simulink model "Active_Suspension_LQR"  (Simulink 7.3)
settings: Solver=ode3  StartTime=0.0  StopTime=50  FixedStep=0.005  RelTol=1e-3
values from neighbouring files (symbols this model uses):
  A = [0,0,-ks/mb,ks/mb,0;0,0,ks/mw,(-kt-ks)/mw,kt/mw;1,0,0,0,0;0,1,0,0,0;0,0,0,0,-2*pi*f0]    [GA_LQR.m]
  B = [1/mb;-1/mw;0;0;0]    [GA_LQR.m]
  C = eye(size(A,1))    [GA_LQR.m]
  D = zeros(size(A,1),size(B,2))    [GA_LQR.m]
  G = [0;0;0;0;2*pi*sqrt(G0*u)]    [GA_LQR.m]
undefined symbols (not defined in the file or in its folder): K
settings Model: Creator=tongji_HEV  LastModifiedBy=tongji_HEV

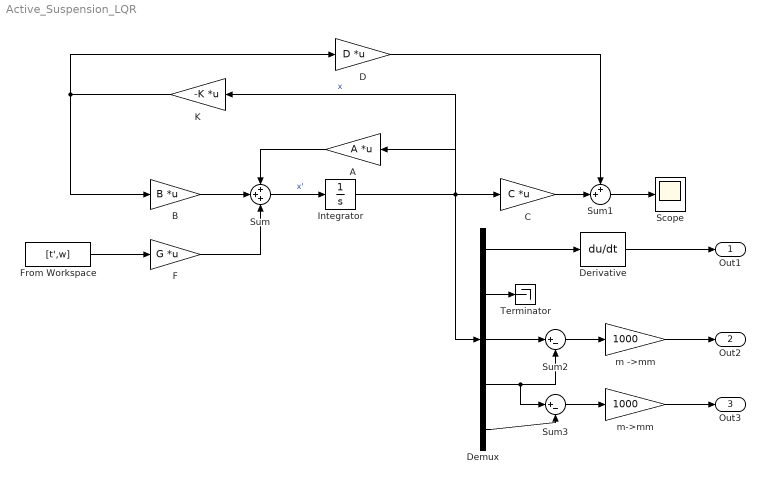
== system Active_Suspension_LQR ==
  A : Gain  Gain=A  Multiplication=Matrix(K*u)  ParameterDataType=fixdt(1, 16)  ParameterScaling=2^0  OutDataType=fixdt(1, 16)  OutScaling=2^0
  B : Gain  Gain=B  Multiplication=Matrix(K*u)  ParameterDataType=fixdt(1, 16)  ParameterScaling=2^0  OutDataType=fixdt(1, 16)  OutScaling=2^0
  C : Gain  Gain=C  Multiplication=Matrix(K*u)  ParameterDataType=fixdt(1, 16)  ParameterScaling=2^0  OutDataType=fixdt(1, 16)  OutScaling=2^0
  D : Gain  Gain=D  Multiplication=Matrix(K*u)  ParameterDataType=fixdt(1, 16)  ParameterScaling=2^0  OutDataType=fixdt(1, 16)  OutScaling=2^0
  Demux : Demux  Outputs=5
  Derivative : Derivative
  F : Gain  Gain=G  Multiplication=Matrix(K*u)  ParameterDataType=fixdt(1, 16)  ParameterScaling=2^0  OutDataType=fixdt(1, 16)  OutScaling=2^0
  From Workspace : FromWorkspace  VariableName=[t',w]  SampleTime=0.005
  Integrator : Integrator
  K : Gain  Gain=-K  Multiplication=Matrix(K*u)  ParameterDataType=fixdt(1, 16)  ParameterScaling=2^0  OutDataType=fixdt(1, 16)  OutScaling=2^0
  Scope : Scope
  Sum : Sum  Inputs=+++  OutDataType=fixdt(1, 16)  OutScaling=2^0
  Sum1 : Sum  Inputs=++|  OutDataType=fixdt(1, 16)  OutScaling=2^0
  Sum2 : Sum  Inputs=|+-  OutDataType=fixdt(1, 16)  OutScaling=2^0
  Sum3 : Sum  Inputs=|+-  OutDataType=fixdt(1, 16)  OutScaling=2^0
  Terminator : Terminator
  m ->mm : Gain  Gain=1000  ParameterDataType=fixdt(1, 16)  ParameterScaling=2^0  OutDataType=fixdt(1, 16)  OutScaling=2^0
  m->mm : Gain  Gain=1000  ParameterDataType=fixdt(1, 16)  ParameterScaling=2^0  OutDataType=fixdt(1, 16)  OutScaling=2^0
  Out1 : Outport  OutDataType=fixdt(1, 16)  OutScaling=2^0
  Out2 : Outport  Port=2  OutDataType=fixdt(1, 16)  OutScaling=2^0
  Out3 : Outport  Port=3  OutDataType=fixdt(1, 16)  OutScaling=2^0
  wires:
  Integrator/1 -> A/1, K/1, C/1, Demux/1  "x"
  Sum/1 -> Integrator/1  "x'"
  D/1 -> Sum1/1
  C/1 -> Sum1/2
  Sum1/1 -> Scope/1
  A/1 -> Sum/1
  B/1 -> Sum/2
  F/1 -> Sum/3
  From Workspace/1 -> F/1
  K/1 -> B/1, D/1
  Demux/1 -> Derivative/1
  Demux/4 -> Sum2/2, Sum3/1
  Demux/5 -> Sum3/2
  Derivative/1 -> Out1/1
  Sum2/1 -> m ->mm/1
  Sum3/1 -> m->mm/1
  Demux/2 -> Terminator/1
  m->mm/1 -> Out3/1
  Demux/3 -> Sum2/1
  m ->mm/1 -> Out2/1
